simulink model "Assignment3"  (R2020b)
settings: Solver=VariableStepAuto  StartTime=0.0  StopTime=10.0  RelTol=1e-3
values from neighbouring files (symbols this model uses):
  Gp = tf(num, den)    [Assignment1.m]    (also in Assignment3.m = tf([2], [2 2 2]); Lecture3_Controllers.m = tf([10], [1 3 4]); Lecture4_DiscretePID.m = tf(Gpn, Gpd))
  Kd = 1/2    (= 0.5)    [Assignment3.m]    (also in Lecture13_PolePlacement.m = -0.05; Lecture4_DiscretePID.m = 0.3)
  Ki = 1/2    (= 0.5)    [Assignment3.m]    (also in Assignment4.m = -K(3); Lecture13_PolePlacement.m = 0.0125; Lecture4_DiscretePID.m = 0.8)
  Kp = 1/2    (= 0.5)    [Assignment3.m]    (also in Lecture13_PolePlacement.m = -0.025; Lecture4_DiscretePID.m = 0.8)
  T = 1/((20*wc)/(2*pi))    (= 0.0010471975512)    [Assignment1.m]    (also in Assignment3.m = [1/(2.5*bw) 1/(10*bw) 1/(25*bw)]; Lecture15_DigitalLSF.m = 1 / ((25 * bandwidth(tf([10], [2 2 1])))); Lecture4_DiscretePID.m = 0.1)
settings Model: Creator=sebastian  LastModifiedBy=sebastian

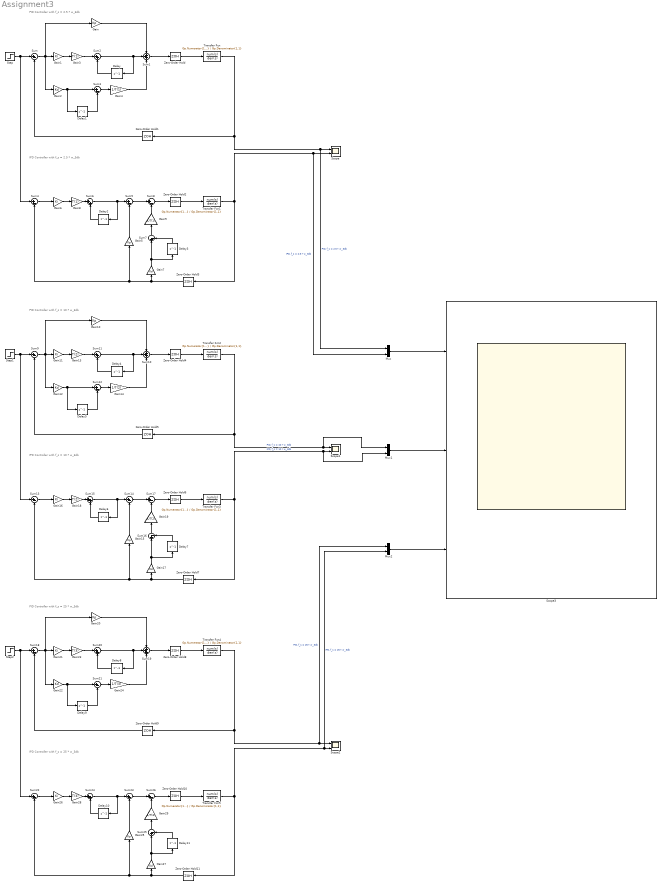
== system Assignment3 ==
  note: PID Controller with f_s = 2.5 * w_3db
  note: IPD Controller with f_s = 2.5 * w_3db
  note: PID Controller with f_s = 10 * w_3db
  note: IPD Controller with f_s = 10 * w_3db
  note: PID Controller with f_s = 25 * w_3db
  note: IPD Controller with f_s = 25 * w_3db
  Delay{,1..3} (4 alike) : Delay  DelayLength=1  SampleTime=T(1)
  Delay{8..11} (4 alike) : Delay  DelayLength=1  SampleTime=T(3)
  Delay{4..7} (4 alike) : Delay  DelayLength=1  SampleTime=T(2)
  Gain{,5,10,15,20,25} (6 alike) : Gain  Gain=Kp
  Gain{1,6,11,16,21,26} (6 alike) : Gain  Gain=Ki
  Gain{2,7,12,17,22,27} (6 alike) : Gain  Gain=Kd
  Gain13 : Gain  Gain=T(2)
  Gain14 : Gain  Gain=1/T(2)
  Gain18 : Gain  Gain=T(2)
  Gain19 : Gain  Gain=1/T(2)
  Gain23 : Gain  Gain=T(3)
  Gain24 : Gain  Gain=1/T(3)
  Gain28 : Gain  Gain=T(3)
  Gain29 : Gain  Gain=1/T(3)
  Gain3 : Gain  Gain=T(1)
  Gain4 : Gain  Gain=1/T(1)
  Gain8 : Gain  Gain=T(1)
  Gain9 : Gain  Gain=1/T(1)
  Mux : Mux  Inputs=2
  Mux1 : Mux  Inputs=2
  Mux2 : Mux  Inputs=2
  Scope : Scope  NumInputPorts=2
  Scope1 : Scope  NumInputPorts=2
  Scope2 : Scope  NumInputPorts=2
  Scope3 : Scope  NumInputPorts=3
  Step : Step  SampleTime=0
  Step1 : Step  SampleTime=0
  Step2 : Step  SampleTime=0
  Sum{,3..5,7..9,12..14,16..18,21..23,25..26} (18 alike) : Sum  Inputs=|+-
  Sum1 : Sum  Inputs=+++
  Sum10 : Sum  Inputs=+++
  Sum{2,6,11,15,20,24} (6 alike) : Sum  Inputs=|++
  Sum19 : Sum  Inputs=+++
  Transfer Fcn{,1..5} (6 alike) : TransferFcn  Numerator=Gp.Numerator{1,1}  Denominator=Gp.Denominator{1,1}
  Zero-Order Hold{,1..3} (4 alike) : ZeroOrderHold  SampleTime=T(1)
  Zero-Order Hold{8..11} (4 alike) : ZeroOrderHold  SampleTime=T(3)
  Zero-Order Hold{4..7} (4 alike) : ZeroOrderHold  SampleTime=T(2)
  wires:
  Gain1/1 -> Gain3/1
  Delay/1 -> Sum2/2
  Gain3/1 -> Sum2/1
  Sum2/1 -> Delay/1, Sum1/2
  Sum/1 -> Gain/1, Gain2/1, Gain1/1
  Gain2/1 -> Delay1/1, Sum3/1
  Delay1/1 -> Sum3/2
  Sum3/1 -> Gain4/1
  Gain4/1 -> Sum1/3
  Gain/1 -> Sum1/1
  Sum1/1 -> Zero-Order Hold/1
  Zero-Order Hold/1 -> Transfer Fcn/1
  Transfer Fcn/1 -> Zero-Order Hold1/1, Mux/1, Scope/1  "PID, f_s = 2.5 * w_3db"
  Zero-Order Hold1/1 -> Sum/2
  Sum4/1 -> Gain6/1
  Gain8/1 -> Sum6/1
  Zero-Order Hold3/1 -> Gain7/1, Gain5/1, Sum4/2
  Transfer Fcn1/1 -> Mux/2, Scope/2, Zero-Order Hold3/1  "IPD, f_s = 2.5 * w_3db"
  Delay2/1 -> Sum6/2
  Sum6/1 -> Sum5/1, Delay2/1
  Step/1 -> Sum4/1, Sum/1
  Zero-Order Hold2/1 -> Transfer Fcn1/1
  Gain6/1 -> Gain8/1
  Gain5/1 -> Sum5/2
  Sum5/1 -> Sum8/1
  Sum8/1 -> Zero-Order Hold2/1
  Gain7/1 -> Delay3/1, Sum7/1
  Delay3/1 -> Sum7/2
  Sum7/1 -> Gain9/1
  Gain9/1 -> Sum8/2
  Sum15/1 -> Sum14/1, Delay6/1
  Sum9/1 -> Gain10/1, Gain12/1, Gain11/1
  Sum14/1 -> Sum17/1
  Gain13/1 -> Sum11/1
  Sum10/1 -> Zero-Order Hold4/1
  Gain19/1 -> Sum17/2
  Sum13/1 -> Gain16/1
  Gain15/1 -> Sum14/2
  Zero-Order Hold6/1 -> Transfer Fcn3/1
  Zero-Order Hold5/1 -> Sum9/2
  Gain17/1 -> Delay7/1, Sum16/1
  Sum11/1 -> Delay4/1, Sum10/2
  Zero-Order Hold7/1 -> Gain17/1, Gain15/1, Sum13/2
  Gain14/1 -> Sum10/3
  Gain16/1 -> Gain18/1
  Transfer Fcn2/1 -> Zero-Order Hold5/1, Mux1/1, Scope1/1  "PID, f_s = 10 * w_3db"
  Sum12/1 -> Gain14/1
  Delay4/1 -> Sum11/2
  Delay5/1 -> Sum12/2
  Delay6/1 -> Sum15/2
  Gain10/1 -> Sum10/1
  Sum17/1 -> Zero-Order Hold6/1
  Sum16/1 -> Gain19/1
  Gain12/1 -> Delay5/1, Sum12/1
  Gain18/1 -> Sum15/1
  Step1/1 -> Sum13/1, Sum9/1
  Zero-Order Hold4/1 -> Transfer Fcn2/1
  Transfer Fcn3/1 -> Mux1/2, Scope1/2, Zero-Order Hold7/1  "IPD, f_s = 10 * w_3db"
  Delay7/1 -> Sum16/2
  Gain11/1 -> Gain13/1
  Sum24/1 -> Sum23/1, Delay10/1
  Sum18/1 -> Gain20/1, Gain22/1, Gain21/1
  Sum23/1 -> Sum26/1
  Gain23/1 -> Sum20/1
  Sum19/1 -> Zero-Order Hold8/1
  Gain29/1 -> Sum26/2
  Sum22/1 -> Gain26/1
  Gain25/1 -> Sum23/2
  Zero-Order Hold10/1 -> Transfer Fcn5/1
  Zero-Order Hold9/1 -> Sum18/2
  Gain27/1 -> Delay11/1, Sum25/1
  Sum20/1 -> Delay8/1, Sum19/2
  Zero-Order Hold11/1 -> Gain27/1, Gain25/1, Sum22/2
  Gain24/1 -> Sum19/3
  Gain26/1 -> Gain28/1
  Transfer Fcn4/1 -> Zero-Order Hold9/1, Mux2/1, Scope2/1  "PID, f_s = 25 * w_3db"
  Sum21/1 -> Gain24/1
  Delay8/1 -> Sum20/2
  Delay9/1 -> Sum21/2
  Delay10/1 -> Sum24/2
  Gain20/1 -> Sum19/1
  Sum26/1 -> Zero-Order Hold10/1
  Sum25/1 -> Gain29/1
  Gain22/1 -> Delay9/1, Sum21/1
  Gain28/1 -> Sum24/1
  Step2/1 -> Sum22/1, Sum18/1
  Zero-Order Hold8/1 -> Transfer Fcn4/1
  Transfer Fcn5/1 -> Mux2/2, Scope2/2, Zero-Order Hold11/1  "IPD, f_s = 25 * w_3db"
  Delay11/1 -> Sum25/2
  Gain21/1 -> Gain23/1
  Mux/1 -> Scope3/1
  Mux1/1 -> Scope3/2
  Mux2/1 -> Scope3/3
